simulink model "triplex_12B_with_contracts"  (R2019b)
settings: Solver=ode3  StartTime=0.0  StopTime=10.0  FixedStep=.1  RelTol=1e-3  EnableMultiTasking=on
model workspace (MAT data in the model file):
  ContractValidatorBlocksMap = containers.Map
  ContractValidatorBlocksMap.serialization.keys = {'triplex_12B/triplex_12B_TriplexSignalMonitorSpec/validator', 'triplex_12B_with_contracts/triplex_12B_TriplexSignalMonitorSpec/validator'}
  ContractValidatorBlocksMap.serialization.values{1}.block = 'triplex_12B/triplex_12B_TriplexSignalMonitorSpec/validator'
  ContractValidatorBlocksMap.serialization.values{1}.assumePorts = 1
  ContractValidatorBlocksMap.serialization.values{1}.guaranteePorts = 6
  ContractValidatorBlocksMap.serialization.values{1}.modeBlocksPorts = 0
  ContractValidatorBlocksMap.serialization.values{1}.portHandles.Inport = [1173.00195312 1174.00195312 1175.00195312 1176.00195312 1177.00195312 1178.00195312 1179.00195312]
  ContractValidatorBlocksMap.serialization.values{1}.portHandles.Outport = 1180.00195312
  ContractValidatorBlocksMap.serialization.values{1}.portHandles.Enable = []
  ContractValidatorBlocksMap.serialization.values{1}.portHandles.Trigger = []
  ContractValidatorBlocksMap.serialization.values{1}.portHandles.State = []
  ContractValidatorBlocksMap.serialization.values{1}.portHandles.LConn = []
  ContractValidatorBlocksMap.serialization.values{1}.portHandles.RConn = []
  ContractValidatorBlocksMap.serialization.values{1}.portHandles.Ifaction = []
  ContractValidatorBlocksMap.serialization.values{1}.portHandles.Reset = []
  ContractValidatorBlocksMap.serialization.values{1}.portConnectivity(1).Type = '1'
  ContractValidatorBlocksMap.serialization.values{1}.portConnectivity(1).Position = [365 -135]
  ContractValidatorBlocksMap.serialization.values{1}.portConnectivity(1).SrcBlock = 5288.00085449
  ContractValidatorBlocksMap.serialization.values{1}.portConnectivity(1).SrcPort = 0
  ContractValidatorBlocksMap.serialization.values{1}.portConnectivity(1).DstBlock = []
  ContractValidatorBlocksMap.serialization.values{1}.portConnectivity(1).DstPort = []
  ContractValidatorBlocksMap.serialization.values{1}.portConnectivity(2).Type = '2'
  ContractValidatorBlocksMap.serialization.values{1}.portConnectivity(2).Position = [365 -65]
  ContractValidatorBlocksMap.serialization.values{1}.portConnectivity(2).SrcBlock = 600.002807617
  ContractValidatorBlocksMap.serialization.values{1}.portConnectivity(2).SrcPort = 0
  ContractValidatorBlocksMap.serialization.values{1}.portConnectivity(2).DstBlock = []
  ContractValidatorBlocksMap.serialization.values{1}.portConnectivity(2).DstPort = []
  ContractValidatorBlocksMap.serialization.values{1}.portConnectivity(3).Type = '3'
  ContractValidatorBlocksMap.serialization.values{1}.portConnectivity(3).Position = [365 5]
  ContractValidatorBlocksMap.serialization.values{1}.portConnectivity(3).SrcBlock = 604.003051758
  ContractValidatorBlocksMap.serialization.values{1}.portConnectivity(3).SrcPort = 0
  ContractValidatorBlocksMap.serialization.values{1}.portConnectivity(3).DstBlock = []
  ContractValidatorBlocksMap.serialization.values{1}.portConnectivity(3).DstPort = []
  ContractValidatorBlocksMap.serialization.values{1}.portConnectivity(4).Type = '4'
  ContractValidatorBlocksMap.serialization.values{1}.portConnectivity(4).Position = [365 75]
  ContractValidatorBlocksMap.serialization.values{1}.portConnectivity(4).SrcBlock = 608.003051758
  ContractValidatorBlocksMap.serialization.values{1}.portConnectivity(4).SrcPort = 0
  ContractValidatorBlocksMap.serialization.values{1}.portConnectivity(4).DstBlock = []
  ContractValidatorBlocksMap.serialization.values{1}.portConnectivity(4).DstPort = []
  ContractValidatorBlocksMap.serialization.values{1}.portConnectivity(5).Type = '5'
  ContractValidatorBlocksMap.serialization.values{1}.portConnectivity(5).Position = [365 145]
  ContractValidatorBlocksMap.serialization.values{1}.portConnectivity(5).SrcBlock = 612.003051758
  ContractValidatorBlocksMap.serialization.values{1}.portConnectivity(5).SrcPort = 0
  ContractValidatorBlocksMap.serialization.values{1}.portConnectivity(5).DstBlock = []
  ContractValidatorBlocksMap.serialization.values{1}.portConnectivity(5).DstPort = []
  ContractValidatorBlocksMap.serialization.values{1}.portConnectivity(6).Type = '6'
  ContractValidatorBlocksMap.serialization.values{1}.portConnectivity(6).Position = [365 215]
  ContractValidatorBlocksMap.serialization.values{1}.portConnectivity(6).SrcBlock = 616.003051758
  ContractValidatorBlocksMap.serialization.values{1}.portConnectivity(6).SrcPort = 0
  ContractValidatorBlocksMap.serialization.values{1}.portConnectivity(6).DstBlock = []
  ContractValidatorBlocksMap.serialization.values{1}.portConnectivity(6).DstPort = []
  ContractValidatorBlocksMap.serialization.values{1}.portConnectivity(7).Type = '7'
  ContractValidatorBlocksMap.serialization.values{1}.portConnectivity(7).Position = [365 285]
  ContractValidatorBlocksMap.serialization.values{1}.portConnectivity(7).SrcBlock = 620.003051758
  ContractValidatorBlocksMap.serialization.values{1}.portConnectivity(7).SrcPort = 0
  ContractValidatorBlocksMap.serialization.values{1}.portConnectivity(7).DstBlock = []
  ContractValidatorBlocksMap.serialization.values{1}.portConnectivity(7).DstPort = []
  ContractValidatorBlocksMap.serialization.values{1}.portConnectivity(8).Type = '1'
  ContractValidatorBlocksMap.serialization.values{1}.portConnectivity(8).Position = [500 75]
  ContractValidatorBlocksMap.serialization.values{1}.portConnectivity(8).SrcBlock = []
  ContractValidatorBlocksMap.serialization.values{1}.portConnectivity(8).SrcPort = []
  ContractValidatorBlocksMap.serialization.values{1}.portConnectivity(8).DstBlock = 884.002807617
  ContractValidatorBlocksMap.serialization.values{1}.portConnectivity(8).DstPort = 0
  ContractValidatorBlocksMap.serialization.values{2}.block = 'triplex_12B_with_contracts/triplex_12B_TriplexSignalMonitorSpec/validator'
  ContractValidatorBlocksMap.serialization.values{2}.assumePorts = 0
  ContractValidatorBlocksMap.serialization.values{2}.guaranteePorts = 6
  ContractValidatorBlocksMap.serialization.values{2}.modeBlocksPorts = 0
  ContractValidatorBlocksMap.serialization.values{2}.portHandles.Inport = [2851.00183105 2852.00195312 2853.00195312 2854.00183105 2855.00195312 2856.00183105]
  ContractValidatorBlocksMap.serialization.values{2}.portHandles.Outport = 2857.00195312
  ContractValidatorBlocksMap.serialization.values{2}.portHandles.Enable = []
  ContractValidatorBlocksMap.serialization.values{2}.portHandles.Trigger = []
  ContractValidatorBlocksMap.serialization.values{2}.portHandles.State = []
  ContractValidatorBlocksMap.serialization.values{2}.portHandles.LConn = []
  ContractValidatorBlocksMap.serialization.values{2}.portHandles.RConn = []
  ContractValidatorBlocksMap.serialization.values{2}.portHandles.Ifaction = []
  ContractValidatorBlocksMap.serialization.values{2}.portHandles.Reset = []
  ContractValidatorBlocksMap.serialization.values{2}.portConnectivity(1).Type = '1'
  ContractValidatorBlocksMap.serialization.values{2}.portConnectivity(1).Position = [14780 -135]
  ContractValidatorBlocksMap.serialization.values{2}.portConnectivity(1).SrcBlock = 1475.00390625
  ContractValidatorBlocksMap.serialization.values{2}.portConnectivity(1).SrcPort = 0
  ContractValidatorBlocksMap.serialization.values{2}.portConnectivity(1).DstBlock = []
  ContractValidatorBlocksMap.serialization.values{2}.portConnectivity(1).DstPort = []
  ContractValidatorBlocksMap.serialization.values{2}.portConnectivity(2).Type = '2'
  ContractValidatorBlocksMap.serialization.values{2}.portConnectivity(2).Position = [14780 -50]
  ContractValidatorBlocksMap.serialization.values{2}.portConnectivity(2).SrcBlock = 1479.00378418
  ContractValidatorBlocksMap.serialization.values{2}.portConnectivity(2).SrcPort = 0
  ContractValidatorBlocksMap.serialization.values{2}.portConnectivity(2).DstBlock = []
  ContractValidatorBlocksMap.serialization.values{2}.portConnectivity(2).DstPort = []
  ContractValidatorBlocksMap.serialization.values{2}.portConnectivity(3).Type = '3'
  ContractValidatorBlocksMap.serialization.values{2}.portConnectivity(3).Position = [14780 35]
  ContractValidatorBlocksMap.serialization.values{2}.portConnectivity(3).SrcBlock = 1483.00402832
  ContractValidatorBlocksMap.serialization.values{2}.portConnectivity(3).SrcPort = 0
  ContractValidatorBlocksMap.serialization.values{2}.portConnectivity(3).DstBlock = []
  ContractValidatorBlocksMap.serialization.values{2}.portConnectivity(3).DstPort = []
  ContractValidatorBlocksMap.serialization.values{2}.portConnectivity(4).Type = '4'
  ContractValidatorBlocksMap.serialization.values{2}.portConnectivity(4).Position = [14780 120]
  ContractValidatorBlocksMap.serialization.values{2}.portConnectivity(4).SrcBlock = 1487.00354004
  ContractValidatorBlocksMap.serialization.values{2}.portConnectivity(4).SrcPort = 0
  ContractValidatorBlocksMap.serialization.values{2}.portConnectivity(4).DstBlock = []
  ContractValidatorBlocksMap.serialization.values{2}.portConnectivity(4).DstPort = []
  ContractValidatorBlocksMap.serialization.values{2}.portConnectivity(5).Type = '5'
  ContractValidatorBlocksMap.serialization.values{2}.portConnectivity(5).Position = [14780 205]
  ContractValidatorBlocksMap.serialization.values{2}.portConnectivity(5).SrcBlock = 1491.00524902
  ContractValidatorBlocksMap.serialization.values{2}.portConnectivity(5).SrcPort = 0
  ContractValidatorBlocksMap.serialization.values{2}.portConnectivity(5).DstBlock = []
  ContractValidatorBlocksMap.serialization.values{2}.portConnectivity(5).DstPort = []
  ContractValidatorBlocksMap.serialization.values{2}.portConnectivity(6).Type = '6'
  ContractValidatorBlocksMap.serialization.values{2}.portConnectivity(6).Position = [14780 290]
  ContractValidatorBlocksMap.serialization.values{2}.portConnectivity(6).SrcBlock = 1495.00378418
  ContractValidatorBlocksMap.serialization.values{2}.portConnectivity(6).SrcPort = 0
  ContractValidatorBlocksMap.serialization.values{2}.portConnectivity(6).DstBlock = []
  ContractValidatorBlocksMap.serialization.values{2}.portConnectivity(6).DstPort = []
  ContractValidatorBlocksMap.serialization.values{2}.portConnectivity(7).Type = '1'
  ContractValidatorBlocksMap.serialization.values{2}.portConnectivity(7).Position = [14915 80]
  ContractValidatorBlocksMap.serialization.values{2}.portConnectivity(7).SrcBlock = []
  ContractValidatorBlocksMap.serialization.values{2}.portConnectivity(7).SrcPort = []
  ContractValidatorBlocksMap.serialization.values{2}.portConnectivity(7).DstBlock = 2601.00195312
  ContractValidatorBlocksMap.serialization.values{2}.portConnectivity(7).DstPort = 0
  ContractValidatorBlocksMap.serialization.uniformity = 0
  ContractValidatorBlocksMap.serialization.keyType = 'char'
  ContractValidatorBlocksMap.serialization.valueType = 'any'
undefined symbols (not defined in the file): contractAfterSimulation, contractBeforeSimulation, ContractBlock, ContractGuaranteeBlock, ContractValidatorBlock, saveValidatorParameters
libraries: cocosimLibs x6
(part 1 of 2)
settings Model: Creator=elliocm  LastModifiedBy=hbourbou
settings DataIOCC: LimitDataPoints=on  SaveFormat=StructureWithTime  SignalLoggingSaveFormat=ModelDataLogs  ReturnWorkspaceOutputs=off
settings OptimizationCC: ExpressionDepthLimit=2147483647  LifeSpan=inf
settings DebuggingCC: UnderspecifiedInitializationDetection=Classic  MergeDetectMultiDrivingBlocksExec=none  SolverPrmCheckMsg=warning  MultiTaskDSMMsg=warning  MultiTaskCondExecSysMsg=none  StateNameClashWarn=warning  SFUnexpectedBacktrackingDiag=warning  SFNoUnconditionalDefaultTransitionDiag=warning  SFExecutionAtInitializationDiag=none  ArithmeticOperatorsInVariantConditions=warning
settings HardwareCC: ProdBitPerPointer=32  ProdBitPerSizeT=32  ProdBitPerPtrDiffT=32  ProdLargestAtomicFloat=None  ProdIntDivRoundTo=Undefined  ProdEndianess=Unspecified  ProdWordSize=32  ProdHWDeviceType=32-bit Generic
settings ModelReferenceCC: PropagateSignalLabelsOutOfModel=off
settings SFSimCC: SimUseLocalCustomCode=off  CustomCodeUndefinedFunction=UseInterfaceOnly
settings RTWCC: RTWUseLocalCustomCode=off
settings CodeAppCC: StateflowObjectComments=on
settings GRTTargetCC: TargetLangStandard=C89/C90 (ANSI)  GeneratePreprocessorConditionals=Disable all
settings ConfigComp: CovMetricSettings=dw  CovHtmlReporting=on  CovSaveCumulativeToWorkspaceVar=on  CovSaveSingleToWorkspaceVar=on  CovExternalEMLEnable=off

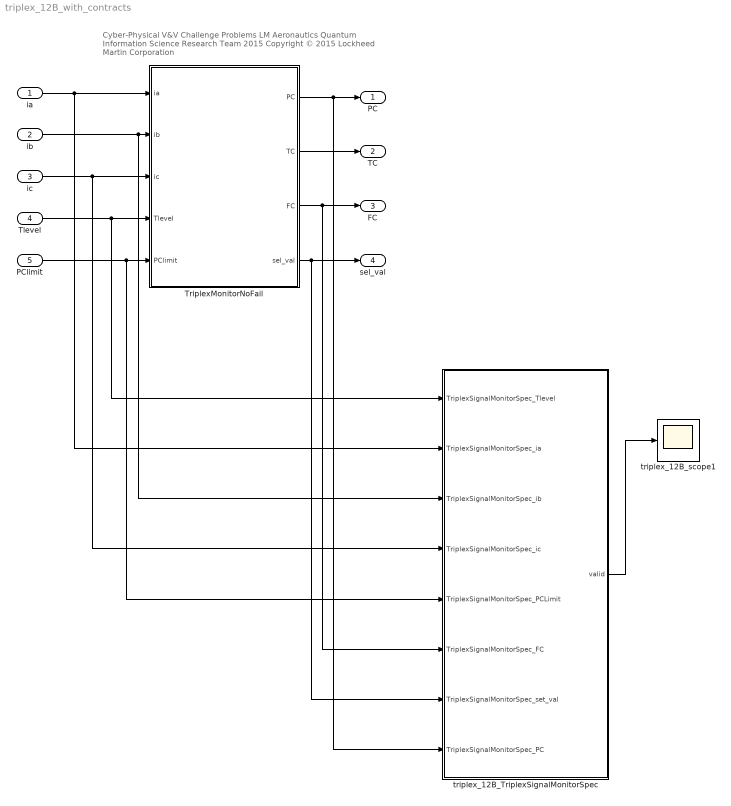
== system triplex_12B_with_contracts ==
  note: Cyber-Physical V&V Challenge Problems
      | LM Aeronautics Quantum Information Science Research Team 2015
      | Copyright © 2015 Lockheed Martin Corporation
  ia : Inport  OutDataTypeStr=double
  ib : Inport  Port=2  OutDataTypeStr=double
  ic : Inport  Port=3  OutDataTypeStr=double
  Tlevel : Inport  Port=4  OutDataTypeStr=double
  PClimit : Inport  Port=5  OutDataTypeStr=int32
  TriplexMonitorNoFail : Subsystem
  triplex_12B_TriplexSignalMonitorSpec : Subsystem  mask(ContractBlock){ContractBlockType=ContractBlock}
      mask init:
      | set_param(gcb, 'LinkStatus', 'none');
      mask DialogControl DescTextVar Prompt: Contract block
      mask Display:
      | text(0.5, 0.5, '{\bf\fontsize{20}Contract}', 'hor', 'center', 'texmode','on');
      | blocks = find_system(gcb, 'LookUnderMasks','all', 'SearchDepth',1,'BlockType','Inport');
      | for i = 1 : length(blocks)
      |     blockName = get_param(blocks(i), 'Name');
      |     [path, blockName] = fileparts(char(blockName));
      |     port_label('input', i, blockName);
      | end
      | 
      | blocks = find_system(gcb, 'LookUnderMasks','all', 'SearchDepth',1,'BlockType','Outport');
      | for i = 1 : length(blocks)
      |     blockName = get_param(blocks(i), 'Name');
      |     [path, blockName] = fileparts(char(blockName));
      |     port_label('output', i, blockName);
      | end
  triplex_12B_scope1 : Scope
  PC : Outport  VectorParamsAs1DForOutWhenUnconnected=off
  TC : Outport  Port=2  VectorParamsAs1DForOutWhenUnconnected=off
  FC : Outport  Port=3  VectorParamsAs1DForOutWhenUnconnected=off
  sel_val : Outport  Port=4  VectorParamsAs1DForOutWhenUnconnected=off
  wires:
  ia/1 -> TriplexMonitorNoFail/1(ia), triplex_12B_TriplexSignalMonitorSpec/2(TriplexSignalMonitorSpec_ia)
  ib/1 -> TriplexMonitorNoFail/2(ib), triplex_12B_TriplexSignalMonitorSpec/3(TriplexSignalMonitorSpec_ib)
  Tlevel/1 -> TriplexMonitorNoFail/4(Tlevel), triplex_12B_TriplexSignalMonitorSpec/1(TriplexSignalMonitorSpec_Tlevel)
  PClimit/1 -> TriplexMonitorNoFail/5(PClimit), triplex_12B_TriplexSignalMonitorSpec/5(TriplexSignalMonitorSpec_PCLimit)
  TriplexMonitorNoFail/2(TC) -> TC/1
  TriplexMonitorNoFail/1(PC) -> PC/1, triplex_12B_TriplexSignalMonitorSpec/8(TriplexSignalMonitorSpec_PC)
  TriplexMonitorNoFail/4(sel_val) -> sel_val/1, triplex_12B_TriplexSignalMonitorSpec/7(TriplexSignalMonitorSpec_set_val)
  ic/1 -> TriplexMonitorNoFail/3(ic), triplex_12B_TriplexSignalMonitorSpec/4(TriplexSignalMonitorSpec_ic)
  TriplexMonitorNoFail/3(FC) -> FC/1, triplex_12B_TriplexSignalMonitorSpec/6(TriplexSignalMonitorSpec_FC)
  triplex_12B_TriplexSignalMonitorSpec/1(valid) -> triplex_12B_scope1/1

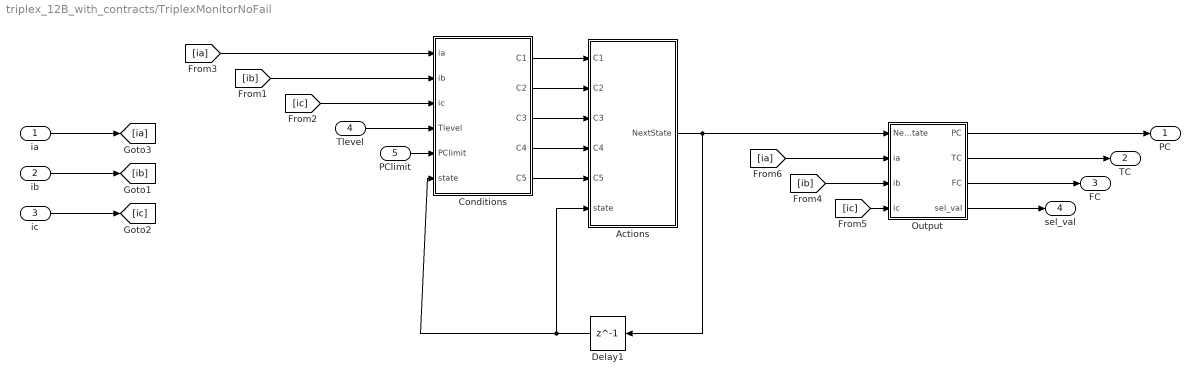
== system triplex_12B_with_contracts/TriplexMonitorNoFail ==
  ia : Inport
  ib : Inport  Port=2
  ic : Inport  Port=3
  Tlevel : Inport  Port=4
  PClimit : Inport  Port=5
  Actions : Subsystem
  Conditions : Subsystem
  Delay1 : Delay  DelayLength=1  InitialCondition=0
  Output : Subsystem
  PC : Outport  VectorParamsAs1DForOutWhenUnconnected=off
  TC : Outport  Port=2  VectorParamsAs1DForOutWhenUnconnected=off
  FC : Outport  Port=3  VectorParamsAs1DForOutWhenUnconnected=off
  sel_val : Outport  Port=4  VectorParamsAs1DForOutWhenUnconnected=off
  wires:
  Conditions/2(C2) -> Actions/2(C2)
  Conditions/5(C5) -> Actions/5(C5)
  Conditions/1(C1) -> Actions/1(C1)
  Conditions/4(C4) -> Actions/4(C4)
  Conditions/3(C3) -> Actions/3(C3)
  Tlevel/1 -> Conditions/4(Tlevel)
  PClimit/1 -> Conditions/5(PClimit)
  Output/2(TC) -> TC/1
  Output/1(PC) -> PC/1
  Output/3(FC) -> FC/1
  Actions/1(NextState) -> Delay1/1, Output/1(NextState)
  Delay1/1 -> Actions/6(state), Conditions/6(state)
  [ia] -> Conditions/1(ia)
  [ib] -> Conditions/2(ib)
  ia/1 -> [ia]
  ib/1 -> [ib]
  ic/1 -> [ic]
  [ic] -> Conditions/3(ic)
  [ia] -> Output/2(ia)
  [ib] -> Output/3(ib)
  [ic] -> Output/4(ic)
  Output/4(sel_val) -> sel_val/1

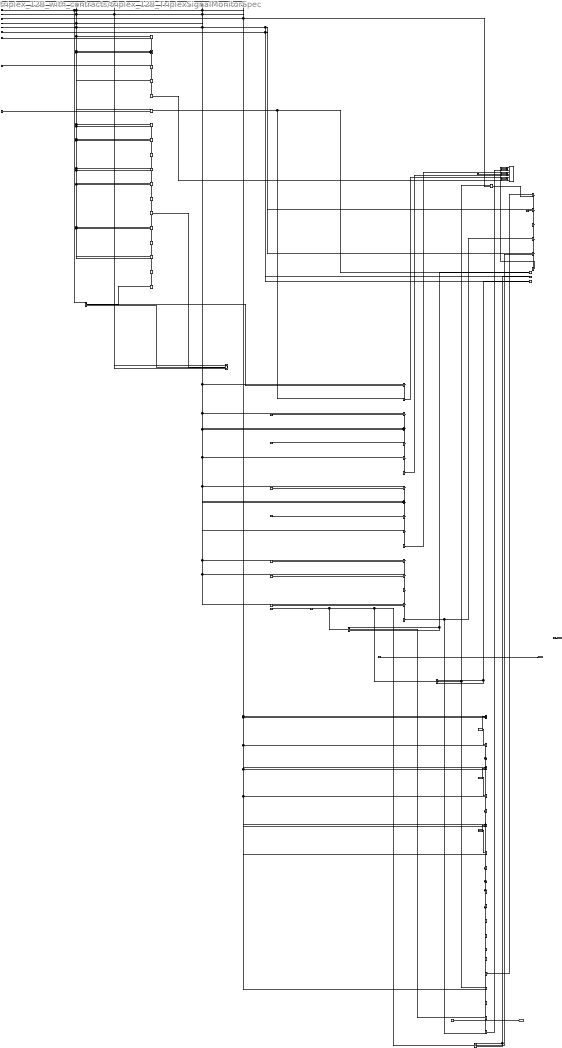
== system triplex_12B_with_contracts/triplex_12B_TriplexSignalMonitorSpec ==
  TriplexSignalMonitorSpec_Tlevel : Inport  OutDataTypeStr=double
  TriplexSignalMonitorSpec_ia : Inport  Port=2  OutDataTypeStr=double
  TriplexSignalMonitorSpec_ib : Inport  Port=3  OutDataTypeStr=double
  TriplexSignalMonitorSpec_ic : Inport  Port=4  OutDataTypeStr=double
  TriplexSignalMonitorSpec_PCLimit : Inport  Port=5
  TriplexSignalMonitorSpec_FC : Inport  Port=6
  TriplexSignalMonitorSpec_set_val : Inport  Port=7  OutDataTypeStr=double
  TriplexSignalMonitorSpec_PC : Inport  Port=8
  Arrow_xxTriplexS_443436564_ec_35_ni_0 : Delay  DelayLength=1  InitialCondition=1
  C1_operator : RelationalOperator  Operator=>  OutDataTypeStr=boolean  RndMeth=Simplest
  C2_operator : RelationalOperator  Operator=>  OutDataTypeStr=boolean  RndMeth=Simplest
  C3_operator : RelationalOperator  Operator=>  OutDataTypeStr=boolean  RndMeth=Simplest
  PRE_xxTriplexSignalMonitorSpec_37 : Delay  DelayLength=1  InitialCondition=0
  PRE_xxTriplexSignalMonitorSpec_40 : Delay  DelayLength=1  InitialCondition=0
  PRE_xxTriplexSignalMonitorSpec_46 : Delay  DelayLength=1  InitialCondition=0
  TSM-001 : Subsystem  mask(ContractGuaranteeBlock){ContractBlockType=ContractGuaranteeBlock}
      mask init:
      | set_param(gcb, 'LinkStatus', 'none');
      mask DialogControl DescTextVar Prompt: Guarantee block
  TSM-002 : Subsystem  mask(ContractGuaranteeBlock){ContractBlockType=ContractGuaranteeBlock}
      mask init:
      | set_param(gcb, 'LinkStatus', 'none');
      mask DialogControl DescTextVar Prompt: Guarantee block
  TSM-003a : Subsystem  mask(ContractGuaranteeBlock){ContractBlockType=ContractGuaranteeBlock}
      mask init:
      | set_param(gcb, 'LinkStatus', 'none');
      mask DialogControl DescTextVar Prompt: Guarantee block
  TSM-003b : Subsystem  mask(ContractGuaranteeBlock){ContractBlockType=ContractGuaranteeBlock}
      mask init:
      | set_param(gcb, 'LinkStatus', 'none');
      mask DialogControl DescTextVar Prompt: Guarantee block
  TSM-003c : Subsystem  mask(ContractGuaranteeBlock){ContractBlockType=ContractGuaranteeBlock}
      mask init:
      | set_param(gcb, 'LinkStatus', 'none');
      mask DialogControl DescTextVar Prompt: Guarantee block
  TSM-004 : Subsystem  mask(ContractGuaranteeBlock){ContractBlockType=ContractGuaranteeBlock}
      mask init:
      | set_param(gcb, 'LinkStatus', 'none');
      mask DialogControl DescTextVar Prompt: Guarantee block
  abs_call : Subsystem
  abs_call1 : Subsystem
  abs_call11 : Subsystem
  branch_10_IF : Switch  Criteria=u2 ~= 0
  branch_11_IF : Switch  Criteria=u2 ~= 0
  branch_12_IF : Switch  Criteria=u2 ~= 0
  branch_13_IF : Switch  Criteria=u2 ~= 0
  branch_9_IF : Switch  Criteria=u2 ~= 0
  failure_in_progress_operator : Logic  AllPortsSameDT=off  OutDataTypeStr=boolean
  failure_must_be_latched_operator : Logic  AllPortsSameDT=off  OutDataTypeStr=boolean
  miscompare_operator : Logic  Operator=OR  AllPortsSameDT=off  OutDataTypeStr=boolean
  no_fail_operator : RelationalOperator  Operator===  OutDataTypeStr=boolean  RndMeth=Simplest
  no_fail_rhs_2 : Constant  Value=0  OutDataTypeStr=int32
  single_fail_reported_operator : Logic  Operator=OR  AllPortsSameDT=off  OutDataTypeStr=boolean
  spec284_operator : cocosimLibs/Implies  SystemSampleTime=-1  Latency=0  AutoFrameSizeCalculation=off
  spec292_operator : cocosimLibs/Implies  SystemSampleTime=-1  Latency=0  AutoFrameSizeCalculation=off
  spec309_operator : cocosimLibs/Implies  SystemSampleTime=-1  Latency=0  AutoFrameSizeCalculation=off
  spec326_operator : cocosimLibs/Implies  SystemSampleTime=-1  Latency=0  AutoFrameSizeCalculation=off
  spec334_operator : cocosimLibs/Implies  SystemSampleTime=-1  Latency=0  AutoFrameSizeCalculation=off
  spec351_operator : cocosimLibs/Implies  SystemSampleTime=-1  Latency=0  AutoFrameSizeCalculation=off
  validator : M-S-Function  LoadFcn=saveValidatorParameters(gcb);  InitFcn=contractBeforeSimulation();  StopFcn=contractAfterSimulation();  FunctionName=contract  mask(ContractValidatorBlock){assumePorts=0, guaranteePorts=6, modePorts=0, ContractBlockType=ContractValidatorBlock, createInportsCheckbox=off}
      mask prompts: assumePorts "Assume ports     :"; guaranteePorts "Guarantee ports :"; modePorts "Mode ports        :"; createInportsCheckbox "Create inports and connect them automatically"
      mask init:
      | set_param(gcb,'LinkStatus','none');
      | contract_callback('inputs_callback',gcb);
      mask DialogControl DescTextVar Prompt: The validator block implements the following logic: <br> <br> <b>Sofar</b>(assume<sub>1</sub> <b>&#8743;</b> assume<sub>2</sub> <b>&#8743;</b> ... assume<sub>k</sub>) <b>&rarr;</b> (guarantee<sub>1</sub> <b>&#8743;</b> guarantee<sub>2</sub> <b>&#8743;</b> ... guarantee<sub>m</sub> <b>&#8743;</b>  mode<sub>1</sub> <b>&#8743;</b> mode<sub>2</sub> <b>&#8743;</b> ... <b>&#8743;</b> mode<sub>n</sub> )<br> where mode<sub>i</sub> = require<sub>i</sub> <b>&rarr;</b> ensure<sub>i</sub>
      mask Display:
      | color('black');
      | port_label('input',1,'guarantee');
      | port_label('input',2,'guarantee');
      | port_label('input',3,'guarantee');
      | port_label('input',4,'guarantee');
      | port_label('input',5,'guarantee');
      | port_label('input',6,'guarantee');
      | port_label('output',1,'valid');
  xxTriplexS_443436564_ec_35_ni_0_init : Constant  Value=0  OutDataTypeStr=boolean
  xxTriplexSignalMonitorSpec_10_operator : Sum  OutDataTypeStr=double
  xxTriplexSignalMonitorSpec_11_operator : Product  OutDataTypeStr=double
  xxTriplexSignalMonitorSpec_11_rhs_1 : Constant  Value=0.5  OutDataTypeStr=double
  xxTriplexSignalMonitorSpec_12_operator : RelationalOperator  Operator===  OutDataTypeStr=boolean  RndMeth=Simplest
  xxTriplexSignalMonitorSpec_13_operator : RelationalOperator  Operator===  OutDataTypeStr=boolean  RndMeth=Simplest
  xxTriplexSignalMonitorSpec_13_rhs_2 : Constant  Value=2  OutDataTypeStr=int32
  xxTriplexSignalMonitorSpec_14_operator : Logic  AllPortsSameDT=off  OutDataTypeStr=boolean
  xxTriplexSignalMonitorSpec_15_operator : RelationalOperator  Operator===  OutDataTypeStr=boolean  RndMeth=Simplest
  xxTriplexSignalMonitorSpec_16_operator : Logic  AllPortsSameDT=off  OutDataTypeStr=boolean
  xxTriplexSignalMonitorSpec_17_operator : Sum  Inputs=+-  OutDataTypeStr=double
  xxTriplexSignalMonitorSpec_19_operator : Sum  Inputs=+-  OutDataTypeStr=double
  xxTriplexSignalMonitorSpec_1_operator : Sum  OutDataTypeStr=double
  xxTriplexSignalMonitorSpec_21_operator : Sum  Inputs=+-  OutDataTypeStr=double
  xxTriplexSignalMonitorSpec_23_operator : RelationalOperator  Operator=<=  OutDataTypeStr=boolean  RndMeth=Simplest
  xxTriplexSignalMonitorSpec_24_operator : RelationalOperator  Operator=<=  OutDataTypeStr=boolean  RndMeth=Simplest
  xxTriplexSignalMonitorSpec_25_operator : Logic  AllPortsSameDT=off  OutDataTypeStr=boolean
  xxTriplexSignalMonitorSpec_26_operator : RelationalOperator  Operator=<=  OutDataTypeStr=boolean  RndMeth=Simplest
  xxTriplexSignalMonitorSpec_27_operator : RelationalOperator  Operator=<=  OutDataTypeStr=boolean  RndMeth=Simplest
  xxTriplexSignalMonitorSpec_28_operator : Logic  AllPortsSameDT=off  OutDataTypeStr=boolean
  xxTriplexSignalMonitorSpec_29_operator : Logic  Operator=OR  AllPortsSameDT=off  OutDataTypeStr=boolean
  xxTriplexSignalMonitorSpec_2_operator : Product  OutDataTypeStr=double
  xxTriplexSignalMonitorSpec_2_rhs_1 : Constant  Value=0.5  OutDataTypeStr=double
  xxTriplexSignalMonitorSpec_30_operator : RelationalOperator  Operator=<=  OutDataTypeStr=boolean  RndMeth=Simplest
  xxTriplexSignalMonitorSpec_31_operator : Logic  AllPortsSameDT=off  OutDataTypeStr=boolean
  xxTriplexSignalMonitorSpec_32_operator : RelationalOperator  Operator=<=  OutDataTypeStr=boolean  RndMeth=Simplest
  xxTriplexSignalMonitorSpec_33_operator : Logic  AllPortsSameDT=off  OutDataTypeStr=boolean
  xxTriplexSignalMonitorSpec_34_operator : Logic  Operator=OR  AllPortsSameDT=off  OutDataTypeStr=boolean
  xxTriplexSignalMonitorSpec_36_rhs : Constant  Value=0  OutDataTypeStr=Inherit: Inherit via back propagation
  xxTriplexSignalMonitorSpec_39_rhs : Constant  Value=0.0  OutDataTypeStr=double
  xxTriplexSignalMonitorSpec_3_operator : RelationalOperator  Operator===  OutDataTypeStr=boolean  RndMeth=Simplest
  xxTriplexSignalMonitorSpec_42_operator : RelationalOperator  Operator=>  OutDataTypeStr=boolean  RndMeth=Simplest
  xxTriplexSignalMonitorSpec_42_rhs_2 : Constant  Value=0  OutDataTypeStr=int32
  xxTriplexSignalMonitorSpec_43_operator : RelationalOperator  Operator=<=  OutDataTypeStr=boolean  RndMeth=Simplest
  xxTriplexSignalMonitorSpec_44_operator : Logic  AllPortsSameDT=off  OutDataTypeStr=boolean
  xxTriplexSignalMonitorSpec_45_operator : RelationalOperator  Operator=>  OutDataTypeStr=boolean  RndMeth=Simplest
  xxTriplexSignalMonitorSpec_47_rhs1 : Constant  Value=true  OutDataTypeStr=boolean
  xxTriplexSignalMonitorSpec_48_operator : RelationalOperator  Operator===  OutDataTypeStr=boolean  RndMeth=Simplest
  xxTriplexSignalMonitorSpec_48_rhs_2 : Constant  Value=4  OutDataTypeStr=int32
  xxTriplexSignalMonitorSpec_49_operator : RelationalOperator  Operator===  OutDataTypeStr=boolean  RndMeth=Simplest
  xxTriplexSignalMonitorSpec_49_rhs_2 : Constant  Value=2  OutDataTypeStr=int32
  xxTriplexSignalMonitorSpec_4_operator : RelationalOperator  Operator===  OutDataTypeStr=boolean  RndMeth=Simplest
  xxTriplexSignalMonitorSpec_4_rhs_2 : Constant  OutDataTypeStr=int32
  xxTriplexSignalMonitorSpec_50_operator : RelationalOperator  Operator===  OutDataTypeStr=boolean  RndMeth=Simplest
  xxTriplexSignalMonitorSpec_50_rhs_2 : Constant  OutDataTypeStr=int32
  xxTriplexSignalMonitorSpec_51_operator : Logic  Operator=OR  AllPortsSameDT=off  OutDataTypeStr=boolean
  xxTriplexSignalMonitorSpec_52_operator : Logic  Operator=NOT  AllPortsSameDT=off  OutDataTypeStr=boolean
  xxTriplexSignalMonitorSpec_53_operator : Logic  AllPortsSameDT=off  OutDataTypeStr=boolean
  xxTriplexSignalMonitorSpec_54_operator : Logic  AllPortsSameDT=off  OutDataTypeStr=boolean
  xxTriplexSignalMonitorSpec_55_operator : Logic  Operator=NOT  AllPortsSameDT=off  OutDataTypeStr=boolean
  xxTriplexSignalMonitorSpec_56_operator : Logic  AllPortsSameDT=off  OutDataTypeStr=boolean
  xxTriplexSignalMonitorSpec_57_operator : Logic  AllPortsSameDT=off  OutDataTypeStr=boolean
  xxTriplexSignalMonitorSpec_58_operator : Logic  Operator=NOT  AllPortsSameDT=off  OutDataTypeStr=boolean
  xxTriplexSignalMonitorSpec_59_operator : Logic  AllPortsSameDT=off  OutDataTypeStr=boolean
  xxTriplexSignalMonitorSpec_5_operator : RelationalOperator  Operator===  OutDataTypeStr=boolean  RndMeth=Simplest
  xxTriplexSignalMonitorSpec_60_operator : Logic  AllPortsSameDT=off  OutDataTypeStr=boolean
  xxTriplexSignalMonitorSpec_61_operator : Logic  Operator=OR  AllPortsSameDT=off  OutDataTypeStr=boolean
  xxTriplexSignalMonitorSpec_6_operator : Sum  OutDataTypeStr=double
  xxTriplexSignalMonitorSpec_7_operator : Product  OutDataTypeStr=double
  xxTriplexSignalMonitorSpec_7_rhs_1 : Constant  Value=0.5  OutDataTypeStr=double
  xxTriplexSignalMonitorSpec_8_operator : RelationalOperator  Operator===  OutDataTypeStr=boolean  RndMeth=Simplest
  xxTriplexSignalMonitorSpec_9_operator : RelationalOperator  Operator===  OutDataTypeStr=boolean  RndMeth=Simplest
  xxTriplexSignalMonitorSpec_9_rhs_2 : Constant  Value=4  OutDataTypeStr=int32
  valid : Outport
  wires:
  validator/1 -> valid/1
  xxTriplexSignalMonitorSpec_9_rhs_2/1 -> xxTriplexSignalMonitorSpec_9_operator/2
  xxTriplexSignalMonitorSpec_7_operator/1 -> xxTriplexSignalMonitorSpec_8_operator/2
  xxTriplexSignalMonitorSpec_6_operator/1 -> xxTriplexSignalMonitorSpec_7_operator/2
  xxTriplexSignalMonitorSpec_7_rhs_1/1 -> xxTriplexSignalMonitorSpec_7_operator/1
  xxTriplexSignalMonitorSpec_57_operator/1 -> xxTriplexSignalMonitorSpec_61_operator/2
  xxTriplexSignalMonitorSpec_60_operator/1 -> xxTriplexSignalMonitorSpec_61_operator/1
  xxTriplexSignalMonitorSpec_59_operator/1 -> xxTriplexSignalMonitorSpec_60_operator/1
  branch_9_IF/1 -> xxTriplexSignalMonitorSpec_5_operator/2
  xxTriplexSignalMonitorSpec_58_operator/1 -> xxTriplexSignalMonitorSpec_59_operator/1
  xxTriplexSignalMonitorSpec_56_operator/1 -> xxTriplexSignalMonitorSpec_57_operator/1
  xxTriplexSignalMonitorSpec_55_operator/1 -> xxTriplexSignalMonitorSpec_56_operator/2
  xxTriplexSignalMonitorSpec_52_operator/1 -> xxTriplexSignalMonitorSpec_54_operator/2
  xxTriplexSignalMonitorSpec_53_operator/1 -> xxTriplexSignalMonitorSpec_54_operator/1
  xxTriplexSignalMonitorSpec_49_operator/1 -> xxTriplexSignalMonitorSpec_51_operator/2
  xxTriplexSignalMonitorSpec_50_operator/1 -> xxTriplexSignalMonitorSpec_51_operator/1
  xxTriplexSignalMonitorSpec_50_rhs_2/1 -> xxTriplexSignalMonitorSpec_50_operator/2
  xxTriplexSignalMonitorSpec_4_rhs_2/1 -> xxTriplexSignalMonitorSpec_4_operator/2
  xxTriplexSignalMonitorSpec_49_rhs_2/1 -> xxTriplexSignalMonitorSpec_49_operator/2
  xxTriplexSignalMonitorSpec_48_rhs_2/1 -> xxTriplexSignalMonitorSpec_48_operator/2
  xxTriplexSignalMonitorSpec_47_rhs1/1 -> [a_e_xxTriplexSignalMonitorSpec_47]
  xxTriplexSignalMonitorSpec_43_operator/1 -> xxTriplexSignalMonitorSpec_44_operator/2
  xxTriplexSignalMonitorSpec_42_rhs_2/1 -> xxTriplexSignalMonitorSpec_42_operator/2
  xxTriplexSignalMonitorSpec_39_rhs/1 -> [a_e_xxTriplexSignalMonitorSpec_41]
  xxTriplexSignalMonitorSpec_2_operator/1 -> xxTriplexSignalMonitorSpec_3_operator/2
  xxTriplexSignalMonitorSpec_36_rhs/1 -> [a_e_xxTriplexSignalMonitorSpec_38]
  xxTriplexSignalMonitorSpec_31_operator/1 -> xxTriplexSignalMonitorSpec_34_operator/2
  xxTriplexSignalMonitorSpec_33_operator/1 -> xxTriplexSignalMonitorSpec_34_operator/1
  xxTriplexSignalMonitorSpec_32_operator/1 -> xxTriplexSignalMonitorSpec_33_operator/2
  xxTriplexSignalMonitorSpec_30_operator/1 -> xxTriplexSignalMonitorSpec_31_operator/1
  xxTriplexSignalMonitorSpec_1_operator/1 -> xxTriplexSignalMonitorSpec_2_operator/2
  xxTriplexSignalMonitorSpec_2_rhs_1/1 -> xxTriplexSignalMonitorSpec_2_operator/1
  xxTriplexSignalMonitorSpec_25_operator/1 -> xxTriplexSignalMonitorSpec_29_operator/2
  xxTriplexSignalMonitorSpec_28_operator/1 -> xxTriplexSignalMonitorSpec_29_operator/1
  xxTriplexSignalMonitorSpec_26_operator/1 -> xxTriplexSignalMonitorSpec_28_operator/2
  xxTriplexSignalMonitorSpec_24_operator/1 -> xxTriplexSignalMonitorSpec_25_operator/1
  failure_in_progress_operator/1 -> xxTriplexSignalMonitorSpec_16_operator/2
  branch_13_IF/1 -> xxTriplexSignalMonitorSpec_15_operator/2
  failure_must_be_latched_operator/1 -> xxTriplexSignalMonitorSpec_14_operator/2
  branch_11_IF/1 -> xxTriplexSignalMonitorSpec_14_operator/1
  xxTriplexSignalMonitorSpec_13_rhs_2/1 -> xxTriplexSignalMonitorSpec_13_operator/2
  xxTriplexSignalMonitorSpec_11_operator/1 -> xxTriplexSignalMonitorSpec_12_operator/2
  xxTriplexSignalMonitorSpec_10_operator/1 -> xxTriplexSignalMonitorSpec_11_operator/2
  xxTriplexSignalMonitorSpec_11_rhs_1/1 -> xxTriplexSignalMonitorSpec_11_operator/1
  TSM-003a/1(guarantee) -> validator/6
  TSM-002/1(guarantee) -> validator/5
  TSM-003c/1(guarantee) -> validator/4
  TSM-003b/1(guarantee) -> validator/3
  TSM-001/1(guarantee) -> validator/2
  TSM-004/1(guarantee) -> validator/1
  xxTriplexSignalMonitorSpec_3_operator/1 -> spec351_operator/2
  xxTriplexSignalMonitorSpec_4_operator/1 -> spec351_operator/1
  xxTriplexSignalMonitorSpec_5_operator/1 -> spec334_operator/2
  xxTriplexSignalMonitorSpec_8_operator/1 -> spec326_operator/2
  xxTriplexSignalMonitorSpec_9_operator/1 -> spec326_operator/1
  xxTriplexSignalMonitorSpec_12_operator/1 -> spec309_operator/2
  xxTriplexSignalMonitorSpec_13_operator/1 -> spec309_operator/1
  xxTriplexSignalMonitorSpec_14_operator/1 -> spec292_operator/1
  xxTriplexSignalMonitorSpec_15_operator/1 -> spec284_operator/2
  xxTriplexSignalMonitorSpec_16_operator/1 -> spec284_operator/1
  xxTriplexSignalMonitorSpec_48_operator/1 -> single_fail_reported_operator/2
  xxTriplexSignalMonitorSpec_51_operator/1 -> single_fail_reported_operator/1
  no_fail_rhs_2/1 -> no_fail_operator/2
  xxTriplexSignalMonitorSpec_54_operator/1 -> miscompare_operator/2
  xxTriplexSignalMonitorSpec_61_operator/1 -> miscompare_operator/1
  spec351_operator/1 -> TSM-003a/1(In1)
  spec334_operator/1 -> TSM-002/1(In1)
  spec326_operator/1 -> TSM-003c/1(In1)
  spec309_operator/1 -> TSM-003b/1(In1)
  spec292_operator/1 -> TSM-001/1(In1)
  spec284_operator/1 -> TSM-004/1(In1)
  xxTriplexSignalMonitorSpec_45_operator/1 -> failure_must_be_latched_operator/2
  xxTriplexSignalMonitorSpec_42_operator/1 -> failure_in_progress_operator/2
  xxTriplexSignalMonitorSpec_44_operator/1 -> failure_in_progress_operator/1
  branch_10_IF/1 -> branch_9_IF/3
  xxTriplexSignalMonitorSpec_29_operator/1 -> branch_9_IF/2
  xxTriplexSignalMonitorSpec_34_operator/1 -> branch_10_IF/2
  xxTriplexSignalMonitorSpec_21_operator/1 -> abs_call11/1(abs_x)
  xxTriplexSignalMonitorSpec_19_operator/1 -> abs_call1/1(abs_x)
  xxTriplexSignalMonitorSpec_17_operator/1 -> abs_call/1(abs_x)
  abs_call11/1(abs_y) -> C3_operator/1
  abs_call1/1(abs_y) -> C2_operator/1
  abs_call/1(abs_y) -> C1_operator/1
  xxTriplexS_443436564_ec_35_ni_0_init/1 -> Arrow_xxTriplexS_443436564_ec_35_ni_0/1
  TriplexSignalMonitorSpec_PC/1 -> xxTriplexSignalMonitorSpec_42_operator/1, PRE_xxTriplexSignalMonitorSpec_37/1
  TriplexSignalMonitorSpec_PCLimit/1 -> xxTriplexSignalMonitorSpec_45_operator/2, xxTriplexSignalMonitorSpec_43_operator/2
  branch_12_IF/1 -> xxTriplexSignalMonitorSpec_45_operator/1, xxTriplexSignalMonitorSpec_43_operator/1
  PRE_xxTriplexSignalMonitorSpec_40/1 -> branch_13_IF/3, branch_13_IF/1
  single_fail_reported_operator/1 -> xxTriplexSignalMonitorSpec_16_operator/1, spec292_operator/2
  miscompare_operator/1 -> xxTriplexSignalMonitorSpec_44_operator/1, failure_must_be_latched_operator/1
  C3_operator/1 -> xxTriplexSignalMonitorSpec_57_operator/2, xxTriplexSignalMonitorSpec_52_operator/1, xxTriplexSignalMonitorSpec_60_operator/2
  C2_operator/1 -> xxTriplexSignalMonitorSpec_55_operator/1, xxTriplexSignalMonitorSpec_53_operator/2, xxTriplexSignalMonitorSpec_59_operator/2
  C1_operator/1 -> xxTriplexSignalMonitorSpec_56_operator/1, xxTriplexSignalMonitorSpec_53_operator/1, xxTriplexSignalMonitorSpec_58_operator/1
  TriplexSignalMonitorSpec_Tlevel/1 -> C3_operator/2, C2_operator/2, C1_operator/2
  PRE_xxTriplexSignalMonitorSpec_37/1 -> branch_12_IF/3, branch_12_IF/1
  Arrow_xxTriplexS_443436564_ec_35_ni_0/1 -> branch_13_IF/2, branch_12_IF/2, branch_11_IF/2
  PRE_xxTriplexSignalMonitorSpec_46/1 -> branch_11_IF/3, branch_11_IF/1
  TriplexSignalMonitorSpec_set_val/1 -> xxTriplexSignalMonitorSpec_8_operator/1, xxTriplexSignalMonitorSpec_12_operator/1, xxTriplexSignalMonitorSpec_5_operator/1, xxTriplexSignalMonitorSpec_15_operator/1, PRE_xxTriplexSignalMonitorSpec_40/1, xxTriplexSignalMonitorSpec_3_operator/1
  no_fail_operator/1 -> spec334_operator/1, PRE_xxTriplexSignalMonitorSpec_46/1
  TriplexSignalMonitorSpec_ia/1 -> xxTriplexSignalMonitorSpec_30_operator/2, xxTriplexSignalMonitorSpec_27_operator/1, xxTriplexSignalMonitorSpec_23_operator/2, xxTriplexSignalMonitorSpec_32_operator/1, xxTriplexSignalMonitorSpec_1_operator/1, xxTriplexSignalMonitorSpec_21_operator/1, xxTriplexSignalMonitorSpec_17_operator/1, xxTriplexSignalMonitorSpec_10_operator/1, branch_10_IF/1
  TriplexSignalMonitorSpec_ib/1 -> xxTriplexSignalMonitorSpec_26_operator/1, xxTriplexSignalMonitorSpec_24_operator/2, xxTriplexSignalMonitorSpec_27_operator/2, xxTriplexSignalMonitorSpec_23_operator/1, xxTriplexSignalMonitorSpec_1_operator/2, xxTriplexSignalMonitorSpec_19_operator/1, xxTriplexSignalMonitorSpec_17_operator/2, xxTriplexSignalMonitorSpec_6_operator/1, branch_9_IF/1
  TriplexSignalMonitorSpec_ic/1 -> xxTriplexSignalMonitorSpec_26_operator/2, xxTriplexSignalMonitorSpec_24_operator/1, xxTriplexSignalMonitorSpec_30_operator/1, xxTriplexSignalMonitorSpec_32_operator/2, xxTriplexSignalMonitorSpec_6_operator/2, xxTriplexSignalMonitorSpec_10_operator/2, xxTriplexSignalMonitorSpec_21_operator/2, xxTriplexSignalMonitorSpec_19_operator/2, branch_10_IF/3
  xxTriplexSignalMonitorSpec_23_operator/1 -> xxTriplexSignalMonitorSpec_33_operator/1, xxTriplexSignalMonitorSpec_25_operator/2
  xxTriplexSignalMonitorSpec_27_operator/1 -> xxTriplexSignalMonitorSpec_31_operator/2, xxTriplexSignalMonitorSpec_28_operator/1
  TriplexSignalMonitorSpec_FC/1 -> xxTriplexSignalMonitorSpec_4_operator/1, no_fail_operator/1, xxTriplexSignalMonitorSpec_49_operator/1, xxTriplexSignalMonitorSpec_48_operator/1, xxTriplexSignalMonitorSpec_50_operator/1, xxTriplexSignalMonitorSpec_13_operator/1, xxTriplexSignalMonitorSpec_9_operator/1

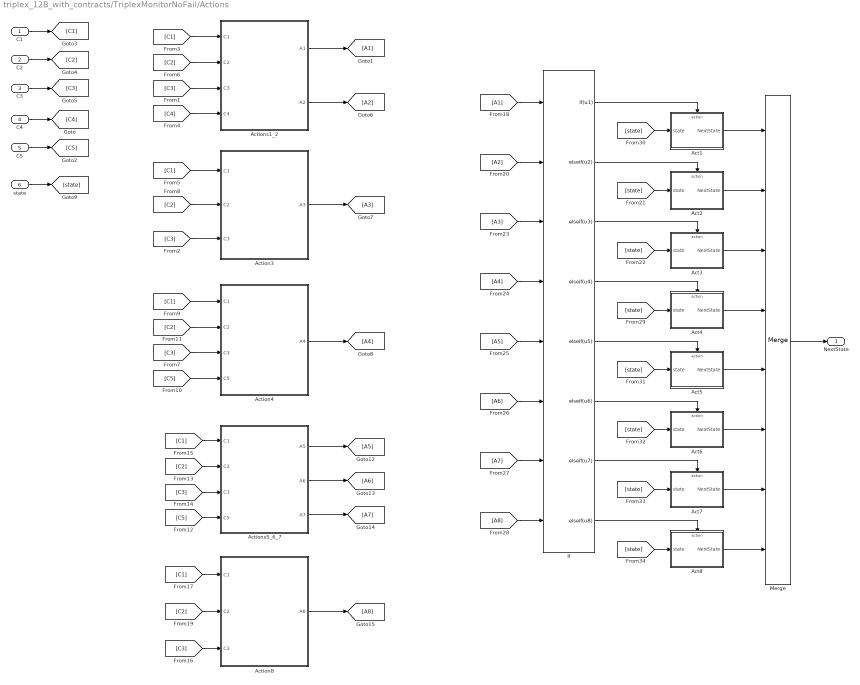
== system triplex_12B_with_contracts/TriplexMonitorNoFail/Actions ==
  C1 : Inport
  C2 : Inport  Port=2
  C3 : Inport  Port=3
  C4 : Inport  Port=4
  C5 : Inport  Port=5
  state : Inport  Port=6
  Act1 : Subsystem
  Act2 : Subsystem
  Act3 : Subsystem
  Act4 : Subsystem
  Act5 : Subsystem
  Act6 : Subsystem
  Act7 : Subsystem
  Act8 : Subsystem
  Action3 : Subsystem
  Action4 : Subsystem
  Action8 : Subsystem
  Actions1_2 : Subsystem
  Actions5_6_7 : Subsystem
  If : If  NumInputs=8  IfExpression=u1  ElseIfExpressions=u2, u3, u4, u5, u6, u7, u8  ShowElse=off
  Merge : Merge  Inputs=8
  NextState : Outport  VectorParamsAs1DForOutWhenUnconnected=off
  wires:
  C1/1 -> [C1]
  C5/1 -> [C5]
  C2/1 -> [C2]
  C3/1 -> [C3]
  C4/1 -> [C4]
  [C1] -> Actions1_2/1(C1)
  [C2] -> Actions1_2/2(C2)
  [C4] -> Actions1_2/4(C4)
  [C3] -> Actions1_2/3(C3)
  Actions1_2/2(A2) -> [A2]
  [C1] -> Action3/1(C1)
  [C2] -> Action3/2(C2)
  [C3] -> Action3/3(C3)
  Action4/1(A4) -> [A4]
  [C1] -> Action4/1(C1)
  [C2] -> Action4/2(C2)
  [C3] -> Action4/3(C3)
  [C5] -> Action4/4(C5)
  [C2] -> Actions5_6_7/2(C2)
  [C3] -> Actions5_6_7/3(C3)
  [C1] -> Actions5_6_7/1(C1)
  [C5] -> Actions5_6_7/4(C5)
  [C1] -> Action8/1(C1)
  [C2] -> Action8/2(C2)
  [C3] -> Action8/3(C3)
  Actions1_2/1(A1) -> [A1]
  Action3/1(A3) -> [A3]
  [A1] -> If/1
  If/1 -> Act1/Action
  [A2] -> If/2
  state/1 -> [state]
  If/2 -> Act2/Action
  If/3 -> Act3/Action
  [A3] -> If/3
  [A4] -> If/4
  [A5] -> If/5
  [A6] -> If/6
  [A7] -> If/7
  [A8] -> If/8
  If/4 -> Act4/Action
  Actions5_6_7/1(A5) -> [A5]
  Actions5_6_7/2(A6) -> [A6]
  Actions5_6_7/3(A7) -> [A7]
  Action8/1(A8) -> [A8]
  [state] -> Act1/1(state)
  If/5 -> Act5/Action
  If/6 -> Act6/Action
  If/7 -> Act7/Action
  If/8 -> Act8/Action
  Act1/1(NextState) -> Merge/1
  Act2/1(NextState) -> Merge/2
  Act3/1(NextState) -> Merge/3
  Act4/1(NextState) -> Merge/4
  Act5/1(NextState) -> Merge/5
  Act6/1(NextState) -> Merge/6
  Act7/1(NextState) -> Merge/7
  Act8/1(NextState) -> Merge/8
  Merge/1 -> NextState/1
  [state] -> Act2/1(state)
  [state] -> Act3/1(state)
  [state] -> Act4/1(state)
  [state] -> Act5/1(state)
  [state] -> Act6/1(state)
  [state] -> Act7/1(state)
  [state] -> Act8/1(state)

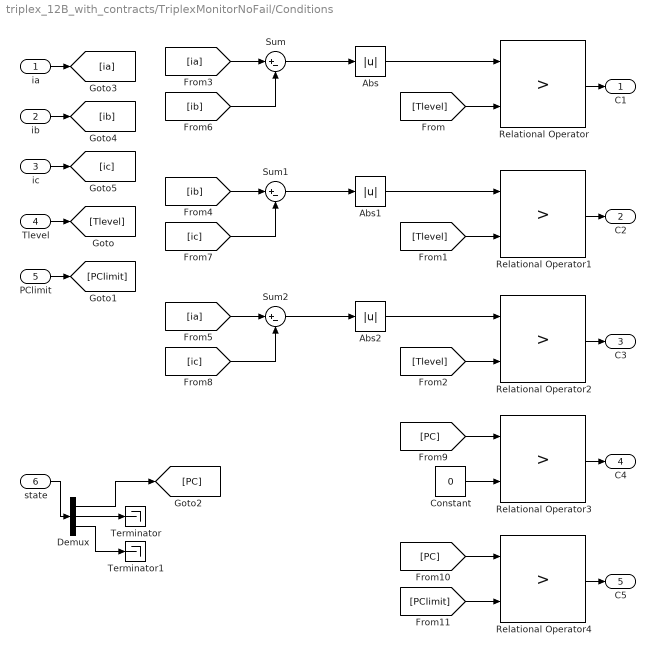
== system triplex_12B_with_contracts/TriplexMonitorNoFail/Conditions ==
  ia : Inport
  ib : Inport  Port=2
  ic : Inport  Port=3
  Tlevel : Inport  Port=4
  PClimit : Inport  Port=5
  state : Inport  Port=6
  Abs : Abs
  Abs1 : Abs
  Abs2 : Abs
  Constant : Constant  Value=0
  Demux : Demux  Outputs=3
  Relational Operator{,1..4} (5 alike) : RelationalOperator  Operator=>  OutDataTypeStr=boolean  RndMeth=Nearest
  Sum : Sum  Inputs=|+-
  Sum1 : Sum  Inputs=|+-
  Sum2 : Sum  Inputs=|+-
  Terminator : Terminator
  Terminator1 : Terminator
  C1 : Outport  VectorParamsAs1DForOutWhenUnconnected=off
  C2 : Outport  Port=2  VectorParamsAs1DForOutWhenUnconnected=off
  C3 : Outport  Port=3  VectorParamsAs1DForOutWhenUnconnected=off
  C4 : Outport  Port=4  VectorParamsAs1DForOutWhenUnconnected=off
  C5 : Outport  Port=5  VectorParamsAs1DForOutWhenUnconnected=off
  wires:
  Abs/1 -> Relational Operator/1
  Sum/1 -> Abs/1
  [Tlevel] -> Relational Operator/2
  Constant/1 -> Relational Operator3/2
  Abs1/1 -> Relational Operator1/1
  [Tlevel] -> Relational Operator1/2
  Sum1/1 -> Abs1/1
  Sum2/1 -> Abs2/1
  Abs2/1 -> Relational Operator2/1
  [Tlevel] -> Relational Operator2/2
  Relational Operator4/1 -> C5/1
  ib/1 -> [ib]
  [ia] -> Sum/1
  Relational Operator1/1 -> C2/1
  [PC] -> Relational Operator4/1
  Tlevel/1 -> [Tlevel]
  [ic] -> Sum1/2
  ia/1 -> [ia]
  ic/1 -> [ic]
  Relational Operator2/1 -> C3/1
  [ic] -> Sum2/2
  [ia] -> Sum2/1
  [ib] -> Sum/2
  [ib] -> Sum1/1
  [PC] -> Relational Operator3/1
  Relational Operator3/1 -> C4/1
  [PClimit] -> Relational Operator4/2
  PClimit/1 -> [PClimit]
  Relational Operator/1 -> C1/1
  state/1 -> Demux/1
  Demux/1 -> [PC]
  Demux/2 -> Terminator/1
  Demux/3 -> Terminator1/1

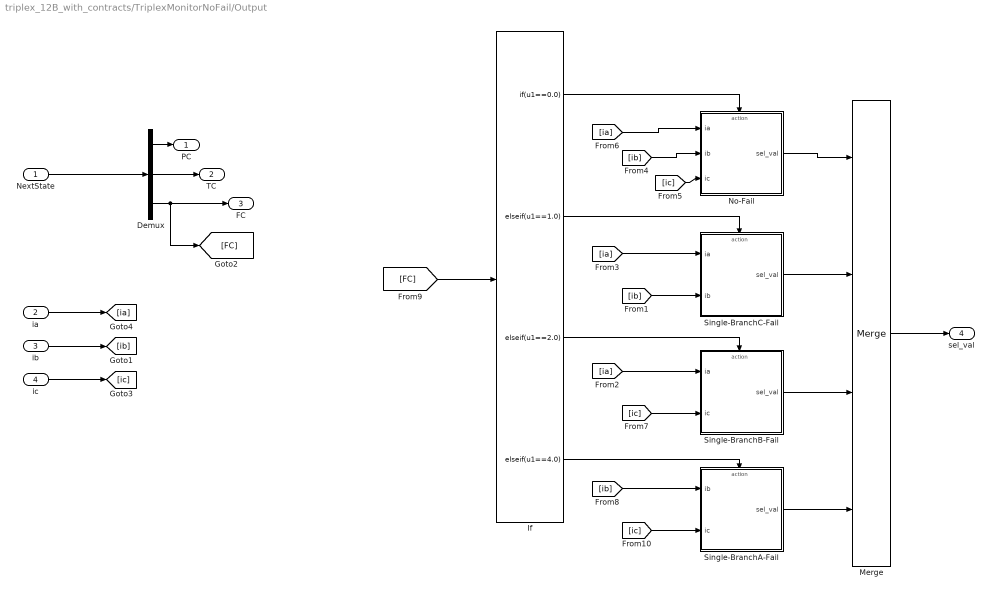
== system triplex_12B_with_contracts/TriplexMonitorNoFail/Output ==
  NextState : Inport
  ia : Inport  Port=2
  ib : Inport  Port=3
  ic : Inport  Port=4
  Demux : Demux  Outputs=3
  If : If  IfExpression=u1==0.0  ElseIfExpressions=u1==1.0, u1==2.0, u1==4.0  ShowElse=off
  Merge : Merge  Inputs=4
  No-Fail : Subsystem
  Single-BranchA-Fail : Subsystem
  Single-BranchB-Fail : Subsystem
  Single-BranchC-Fail : Subsystem
  PC : Outport  VectorParamsAs1DForOutWhenUnconnected=off
  TC : Outport  Port=2  VectorParamsAs1DForOutWhenUnconnected=off
  FC : Outport  Port=3  VectorParamsAs1DForOutWhenUnconnected=off
  sel_val : Outport  Port=4  VectorParamsAs1DForOutWhenUnconnected=off
  wires:
  NextState/1 -> Demux/1
  Demux/1 -> PC/1
  Demux/2 -> TC/1
  Demux/3 -> [FC], FC/1
  [FC] -> If/1
  If/1 -> No-Fail/Action
  ia/1 -> [ia]
  ib/1 -> [ib]
  ic/1 -> [ic]
  Merge/1 -> sel_val/1
  [ia] -> No-Fail/1(ia)
  [ib] -> No-Fail/2(ib)
  [ic] -> No-Fail/3(ic)
  If/2 -> Single-BranchC-Fail/Action
  [ia] -> Single-BranchC-Fail/1(ia)
  [ib] -> Single-BranchC-Fail/2(ib)
  If/3 -> Single-BranchB-Fail/Action
  [ia] -> Single-BranchB-Fail/1(ia)
  [ic] -> Single-BranchB-Fail/2(ic)
  If/4 -> Single-BranchA-Fail/Action
  [ib] -> Single-BranchA-Fail/1(ib)
  [ic] -> Single-BranchA-Fail/2(ic)
  No-Fail/1(sel_val) -> Merge/1
  Single-BranchC-Fail/1(sel_val) -> Merge/2
  Single-BranchB-Fail/1(sel_val) -> Merge/3
  Single-BranchA-Fail/1(sel_val) -> Merge/4

== system triplex_12B_with_contracts/triplex_12B_TriplexSignalMonitorSpec/TSM-001 ==
  In1 : Inport
  guarantee : Outport  OutDataTypeStr=boolean
  wires:
  In1/1 -> guarantee/1

== system triplex_12B_with_contracts/triplex_12B_TriplexSignalMonitorSpec/TSM-002 ==
  In1 : Inport
  guarantee : Outport  OutDataTypeStr=boolean
  wires:
  In1/1 -> guarantee/1

== system triplex_12B_with_contracts/triplex_12B_TriplexSignalMonitorSpec/TSM-003a ==
  In1 : Inport
  guarantee : Outport  OutDataTypeStr=boolean
  wires:
  In1/1 -> guarantee/1

== system triplex_12B_with_contracts/triplex_12B_TriplexSignalMonitorSpec/TSM-003b ==
  In1 : Inport
  guarantee : Outport  OutDataTypeStr=boolean
  wires:
  In1/1 -> guarantee/1

== system triplex_12B_with_contracts/triplex_12B_TriplexSignalMonitorSpec/TSM-003c ==
  In1 : Inport
  guarantee : Outport  OutDataTypeStr=boolean
  wires:
  In1/1 -> guarantee/1

== system triplex_12B_with_contracts/triplex_12B_TriplexSignalMonitorSpec/TSM-004 ==
  In1 : Inport
  guarantee : Outport  OutDataTypeStr=boolean
  wires:
  In1/1 -> guarantee/1

== system triplex_12B_with_contracts/triplex_12B_TriplexSignalMonitorSpec/abs_call ==
  abs_x : Inport  OutDataTypeStr=double
  branch_6_IF : Switch  Criteria=u2 ~= 0
  xxabs_1_operator : RelationalOperator  OutDataTypeStr=boolean  RndMeth=Simplest
  xxabs_1_rhs_2 : Constant  Value=0.0  OutDataTypeStr=double
  xxabs_2_operator : Gain  Gain=-1  OutDataTypeStr=double
  abs_y : Outport
  wires:
  branch_6_IF/1 -> abs_y/1
  xxabs_1_rhs_2/1 -> xxabs_1_operator/2
  xxabs_2_operator/1 -> branch_6_IF/3
  xxabs_1_operator/1 -> branch_6_IF/2
  abs_x/1 -> xxabs_2_operator/1, xxabs_1_operator/1, branch_6_IF/1

== system triplex_12B_with_contracts/triplex_12B_TriplexSignalMonitorSpec/abs_call1 ==
  abs_x : Inport  OutDataTypeStr=double
  branch_6_IF : Switch  Criteria=u2 ~= 0
  xxabs_1_operator : RelationalOperator  OutDataTypeStr=boolean  RndMeth=Simplest
  xxabs_1_rhs_2 : Constant  Value=0.0  OutDataTypeStr=double
  xxabs_2_operator : Gain  Gain=-1  OutDataTypeStr=double
  abs_y : Outport
  wires:
  branch_6_IF/1 -> abs_y/1
  xxabs_1_rhs_2/1 -> xxabs_1_operator/2
  xxabs_2_operator/1 -> branch_6_IF/3
  xxabs_1_operator/1 -> branch_6_IF/2
  abs_x/1 -> xxabs_2_operator/1, xxabs_1_operator/1, branch_6_IF/1

== system triplex_12B_with_contracts/triplex_12B_TriplexSignalMonitorSpec/abs_call11 ==
  abs_x : Inport  OutDataTypeStr=double
  branch_6_IF : Switch  Criteria=u2 ~= 0
  xxabs_1_operator : RelationalOperator  OutDataTypeStr=boolean  RndMeth=Simplest
  xxabs_1_rhs_2 : Constant  Value=0.0  OutDataTypeStr=double
  xxabs_2_operator : Gain  Gain=-1  OutDataTypeStr=double
  abs_y : Outport
  wires:
  branch_6_IF/1 -> abs_y/1
  xxabs_1_rhs_2/1 -> xxabs_1_operator/2
  xxabs_2_operator/1 -> branch_6_IF/3
  xxabs_1_operator/1 -> branch_6_IF/2
  abs_x/1 -> xxabs_2_operator/1, xxabs_1_operator/1, branch_6_IF/1

== system triplex_12B_with_contracts/TriplexMonitorNoFail/Actions/Act1 ==
  note: // Action 1: No pending failures
  state : Inport
  Action Port : ActionPort  ActionPortLabel=if { }
  Constant1 : Constant  Value=0  OutDataTypeStr=int32
  Demux : Demux  Outputs=3
  Mux : Mux  Inputs=3
  Signal Conversion : SignalConversion  OverrideOpt=off
  Terminator : Terminator
  NextState : Outport  VectorParamsAs1DForOutWhenUnconnected=off
  wires:
  state/1 -> [state]
  Signal Conversion/1 -> NextState/1
  Mux/1 -> Signal Conversion/1
  [state] -> Demux/1
  Demux/2 -> Mux/2
  Demux/3 -> Mux/3
  Constant1/1 -> Mux/1
  Demux/1 -> Terminator/1

== system triplex_12B_with_contracts/TriplexMonitorNoFail/Actions/Act2 ==
  note: // Action 2: Failure pending but no miscompares
  state : Inport
  Action Port : ActionPort  ActionPortLabel=elseif { }
  Constant1 : Constant  OutDataTypeStr=int32
  Demux : Demux  Outputs=3
  Mux : Mux  Inputs=3
  Signal Conversion : SignalConversion  OverrideOpt=off
  Sum : Sum  Inputs=-+|
  NextState : Outport  VectorParamsAs1DForOutWhenUnconnected=off
  wires:
  state/1 -> [state]
  Constant1/1 -> Sum/1
  Signal Conversion/1 -> NextState/1
  Mux/1 -> Signal Conversion/1
  [state] -> Demux/1
  Demux/2 -> Mux/2
  Demux/3 -> Mux/3
  Sum/1 -> Mux/1
  Demux/1 -> Sum/2

== system triplex_12B_with_contracts/TriplexMonitorNoFail/Actions/Act3 ==
  note: // Action 3: Do nothing there is only 1 miscompare
  state : Inport
  Action Port : ActionPort  ActionPortLabel=elseif { }
  NextState : Outport  VectorParamsAs1DForOutWhenUnconnected=off
  wires:
  state/1 -> NextState/1

== system triplex_12B_with_contracts/TriplexMonitorNoFail/Actions/Act4 ==
  note: // Action 4: Failure pending
  state : Inport
  Action Port : ActionPort  ActionPortLabel=elseif { }
  Constant1 : Constant  OutDataTypeStr=int32
  Demux : Demux  Outputs=3
  Mux : Mux  Inputs=3
  Signal Conversion : SignalConversion  OverrideOpt=off
  Sum : Sum  Inputs=++|
  Sum1 : Sum  Inputs=|++
  NextState : Outport  VectorParamsAs1DForOutWhenUnconnected=off
  wires:
  state/1 -> [state]
  Signal Conversion/1 -> NextState/1
  Mux/1 -> Signal Conversion/1
  [state] -> Demux/1
  Demux/2 -> Sum/2
  Constant1/1 -> Sum1/2, Sum/1
  Demux/1 -> Sum1/1
  Sum1/1 -> Mux/1
  Sum/1 -> Mux/2
  Demux/3 -> Mux/3

== system triplex_12B_with_contracts/TriplexMonitorNoFail/Actions/Act5 ==
  note: // Action 5: Failure latched (branch B)
  state : Inport
  Action Port : ActionPort  ActionPortLabel=elseif { }
  Constant : Constant  Value=0  OutDataTypeStr=int32
  Constant1 : Constant  Value=2  OutDataTypeStr=int32
  Mux : Mux  Inputs=3
  Selector : Selector  InputPortWidth=3  IndexOptions=Index vector (dialog)  Indices=[2]  OutputSizes=1
  Signal Conversion : SignalConversion  OverrideOpt=off
  NextState : Outport  VectorParamsAs1DForOutWhenUnconnected=off
  wires:
  state/1 -> [state]
  Mux/1 -> Signal Conversion/1
  Constant/1 -> Mux/1
  Constant1/1 -> Mux/3
  Selector/1 -> Mux/2
  [state] -> Selector/1
  Signal Conversion/1 -> NextState/1

== system triplex_12B_with_contracts/TriplexMonitorNoFail/Actions/Act6 ==
  note: // Action 6: Failure latched (branch A)
  state : Inport
  Action Port : ActionPort  ActionPortLabel=elseif { }
  Constant : Constant  Value=0  OutDataTypeStr=int32
  Constant1 : Constant  Value=4  OutDataTypeStr=int32
  Mux : Mux  Inputs=3
  Selector : Selector  InputPortWidth=3  IndexOptions=Index vector (dialog)  Indices=[2]  OutputSizes=1
  Signal Conversion : SignalConversion  OverrideOpt=off
  NextState : Outport  VectorParamsAs1DForOutWhenUnconnected=off
  wires:
  state/1 -> [state]
  Mux/1 -> Signal Conversion/1
  Constant/1 -> Mux/1
  Constant1/1 -> Mux/3
  Selector/1 -> Mux/2
  [state] -> Selector/1
  Signal Conversion/1 -> NextState/1

== system triplex_12B_with_contracts/TriplexMonitorNoFail/Actions/Act7 ==
  note: /// Action 7: Failure latched (branch C)
  state : Inport
  Action Port : ActionPort  ActionPortLabel=elseif { }
  Constant : Constant  Value=0  OutDataTypeStr=int32
  Constant1 : Constant  OutDataTypeStr=int32
  Mux : Mux  Inputs=3
  Selector : Selector  InputPortWidth=3  IndexOptions=Index vector (dialog)  Indices=[2]  OutputSizes=1
  Signal Conversion : SignalConversion  OverrideOpt=off
  NextState : Outport  VectorParamsAs1DForOutWhenUnconnected=off
  wires:
  state/1 -> [state]
  Mux/1 -> Signal Conversion/1
  Constant/1 -> Mux/1
  Constant1/1 -> Mux/3
  Selector/1 -> Mux/2
  [state] -> Selector/1
  Signal Conversion/1 -> NextState/1

== system triplex_12B_with_contracts/TriplexMonitorNoFail/Actions/Act8 ==
  note: // Action 8: All branches miscompare
  state : Inport
  Action Port : ActionPort  ActionPortLabel=elseif { }
  Constant1 : Constant  OutDataTypeStr=int32
  Demux : Demux  Outputs=3
  Mux : Mux  Inputs=3
  Signal Conversion : SignalConversion  OverrideOpt=off
  Sum1 : Sum  Inputs=++|
  NextState : Outport  VectorParamsAs1DForOutWhenUnconnected=off
  wires:
  state/1 -> [state]
  Mux/1 -> Signal Conversion/1
  Demux/1 -> Mux/1
  Demux/3 -> Mux/3
  Sum1/1 -> Mux/2
  Constant1/1 -> Sum1/1
  Demux/2 -> Sum1/2
  Signal Conversion/1 -> NextState/1
  [state] -> Demux/1

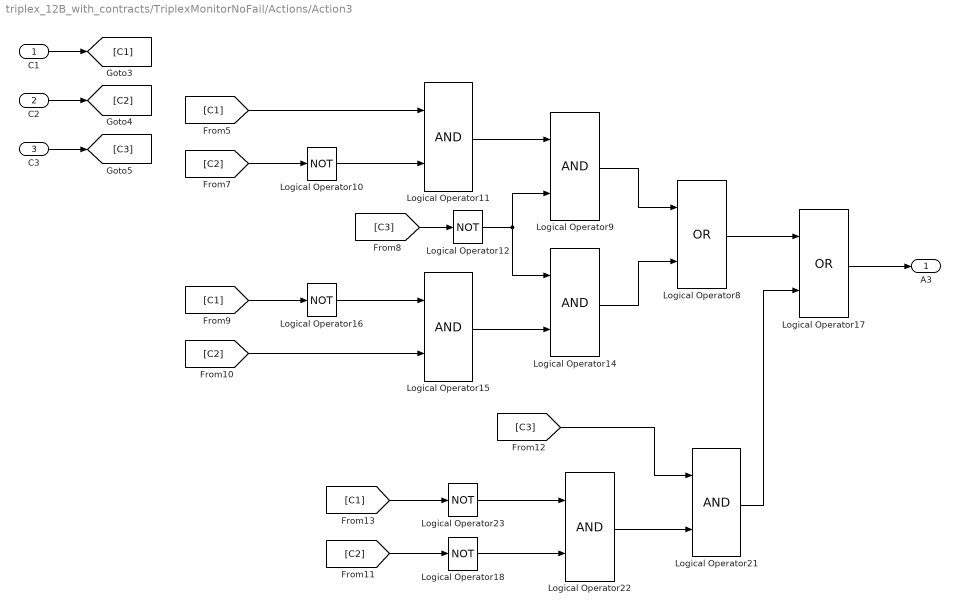
== system triplex_12B_with_contracts/TriplexMonitorNoFail/Actions/Action3 ==
  C1 : Inport
  C2 : Inport  Port=2
  C3 : Inport  Port=3
  Logical Operator{10,12,16,18,23} (5 alike) : Logic  Operator=NOT  Inputs=1  AllPortsSameDT=off  OutDataTypeStr=boolean
  Logical Operator{9,11,14..15,21..22} (6 alike) : Logic  AllPortsSameDT=off  OutDataTypeStr=boolean
  Logical Operator17 : Logic  Operator=OR  AllPortsSameDT=off  OutDataTypeStr=boolean
  Logical Operator8 : Logic  Operator=OR  AllPortsSameDT=off  OutDataTypeStr=boolean
  A3 : Outport  VectorParamsAs1DForOutWhenUnconnected=off
  wires:
  [C1] -> Logical Operator11/1
  [C2] -> Logical Operator10/1
  Logical Operator10/1 -> Logical Operator11/2
  Logical Operator12/1 -> Logical Operator9/2, Logical Operator14/1
  [C3] -> Logical Operator12/1
  Logical Operator11/1 -> Logical Operator9/1
  Logical Operator16/1 -> Logical Operator15/1
  [C1] -> Logical Operator16/1
  Logical Operator9/1 -> Logical Operator8/1
  [C2] -> Logical Operator15/2
  Logical Operator15/1 -> Logical Operator14/2
  Logical Operator14/1 -> Logical Operator8/2
  Logical Operator8/1 -> Logical Operator17/1
  Logical Operator21/1 -> Logical Operator17/2
  [C2] -> Logical Operator18/1
  [C1] -> Logical Operator23/1
  [C3] -> Logical Operator21/1
  Logical Operator23/1 -> Logical Operator22/1
  Logical Operator22/1 -> Logical Operator21/2
  Logical Operator18/1 -> Logical Operator22/2
  Logical Operator17/1 -> A3/1
  C1/1 -> [C1]
  C2/1 -> [C2]
  C3/1 -> [C3]

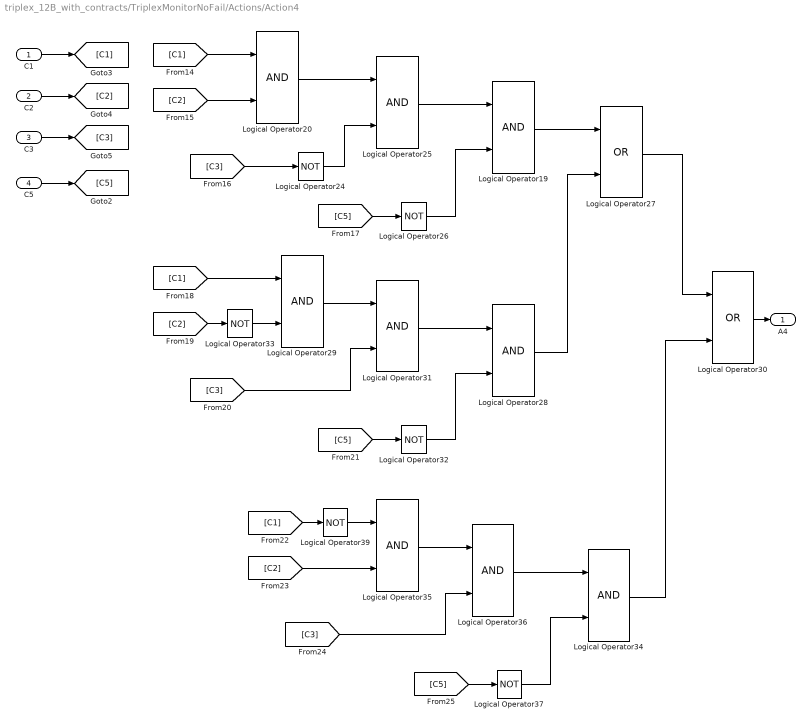
== system triplex_12B_with_contracts/TriplexMonitorNoFail/Actions/Action4 ==
  C1 : Inport
  C2 : Inport  Port=2
  C3 : Inport  Port=3
  C5 : Inport  Port=4
  Logical Operator{19..20,25,28..29,31,34..36} (9 alike) : Logic  AllPortsSameDT=off  OutDataTypeStr=boolean
  Logical Operator{24,26,32..33,37,39} (6 alike) : Logic  Operator=NOT  Inputs=1  AllPortsSameDT=off  OutDataTypeStr=boolean
  Logical Operator27 : Logic  Operator=OR  AllPortsSameDT=off  OutDataTypeStr=boolean
  Logical Operator30 : Logic  Operator=OR  AllPortsSameDT=off  OutDataTypeStr=boolean
  A4 : Outport  VectorParamsAs1DForOutWhenUnconnected=off
  wires:
  [C3] -> Logical Operator31/2
  Logical Operator31/1 -> Logical Operator28/1
  [C5] -> Logical Operator32/1
  Logical Operator32/1 -> Logical Operator28/2
  [C1] -> Logical Operator29/1
  Logical Operator28/1 -> Logical Operator27/2
  Logical Operator29/1 -> Logical Operator31/1
  [C2] -> Logical Operator33/1
  [C3] -> Logical Operator24/1
  [C2] -> Logical Operator20/2
  [C1] -> Logical Operator20/1
  Logical Operator20/1 -> Logical Operator25/1
  Logical Operator30/1 -> A4/1
  Logical Operator26/1 -> Logical Operator19/2
  Logical Operator33/1 -> Logical Operator29/2
  Logical Operator25/1 -> Logical Operator19/1
  [C5] -> Logical Operator26/1
  Logical Operator19/1 -> Logical Operator27/1
  Logical Operator24/1 -> Logical Operator25/2
  Logical Operator36/1 -> Logical Operator34/1
  Logical Operator27/1 -> Logical Operator30/1
  Logical Operator37/1 -> Logical Operator34/2
  [C5] -> Logical Operator37/1
  [C3] -> Logical Operator36/2
  Logical Operator39/1 -> Logical Operator35/1
  Logical Operator35/1 -> Logical Operator36/1
  [C1] -> Logical Operator39/1
  Logical Operator34/1 -> Logical Operator30/2
  [C2] -> Logical Operator35/2
  C1/1 -> [C1]
  C5/1 -> [C5]
  C2/1 -> [C2]
  C3/1 -> [C3]

== system triplex_12B_with_contracts/TriplexMonitorNoFail/Actions/Action8 ==
  C1 : Inport
  C2 : Inport  Port=2
  C3 : Inport  Port=3
  Logical Operator3 : Logic  AllPortsSameDT=off  OutDataTypeStr=boolean
  Logical Operator4 : Logic  AllPortsSameDT=off  OutDataTypeStr=boolean
  A8 : Outport  VectorParamsAs1DForOutWhenUnconnected=off
  wires:
  Logical Operator3/1 -> Logical Operator4/1
  C3/1 -> Logical Operator4/2
  C1/1 -> Logical Operator3/1
  C2/1 -> Logical Operator3/2
  Logical Operator4/1 -> A8/1

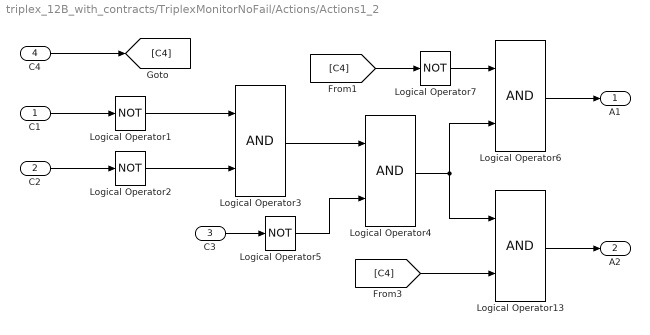
== system triplex_12B_with_contracts/TriplexMonitorNoFail/Actions/Actions1_2 ==
  C1 : Inport
  C2 : Inport  Port=2
  C3 : Inport  Port=3
  C4 : Inport  Port=4
  Logical Operator{1..2,5,7} (4 alike) : Logic  Operator=NOT  Inputs=1  AllPortsSameDT=off  OutDataTypeStr=boolean
  Logical Operator{3..4,6,13} (4 alike) : Logic  AllPortsSameDT=off  OutDataTypeStr=boolean
  A1 : Outport  VectorParamsAs1DForOutWhenUnconnected=off
  A2 : Outport  Port=2  VectorParamsAs1DForOutWhenUnconnected=off
  wires:
  C2/1 -> Logical Operator2/1
  Logical Operator4/1 -> Logical Operator6/2, Logical Operator13/1
  Logical Operator2/1 -> Logical Operator3/2
  [C4] -> Logical Operator13/2
  C1/1 -> Logical Operator1/1
  Logical Operator1/1 -> Logical Operator3/1
  Logical Operator6/1 -> A1/1
  Logical Operator7/1 -> Logical Operator6/1
  Logical Operator3/1 -> Logical Operator4/1
  [C4] -> Logical Operator7/1
  Logical Operator13/1 -> A2/1
  Logical Operator5/1 -> Logical Operator4/2
  C3/1 -> Logical Operator5/1
  C4/1 -> [C4]

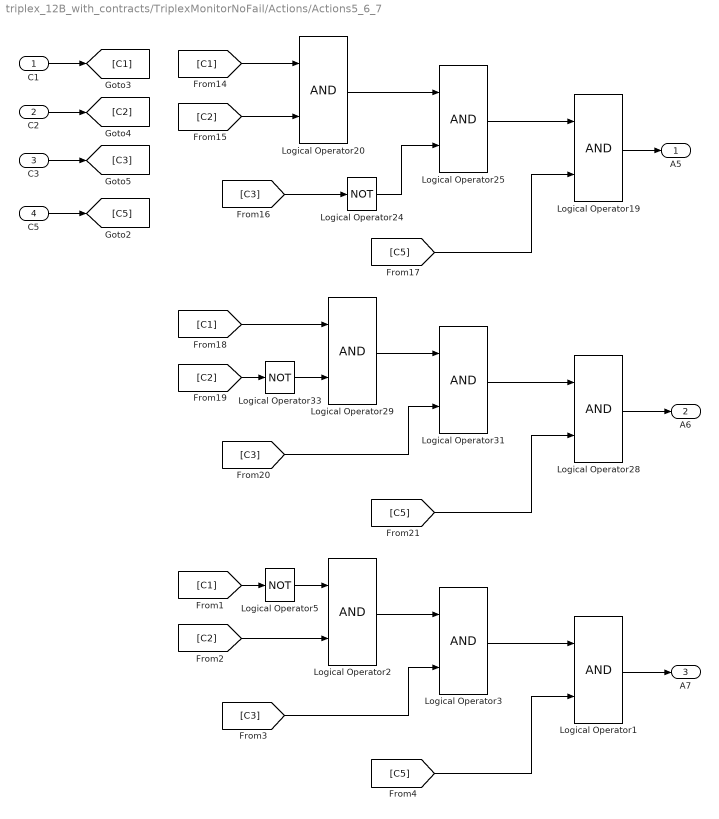
== system triplex_12B_with_contracts/TriplexMonitorNoFail/Actions/Actions5_6_7 ==
  C1 : Inport
  C2 : Inport  Port=2
  C3 : Inport  Port=3
  C5 : Inport  Port=4
  Logical Operator{1..3,19..20,25,28..29,31} (9 alike) : Logic  AllPortsSameDT=off  OutDataTypeStr=boolean
  Logical Operator24 : Logic  Operator=NOT  Inputs=1  AllPortsSameDT=off  OutDataTypeStr=boolean
  Logical Operator33 : Logic  Operator=NOT  Inputs=1  AllPortsSameDT=off  OutDataTypeStr=boolean
  Logical Operator5 : Logic  Operator=NOT  Inputs=1  AllPortsSameDT=off  OutDataTypeStr=boolean
  A5 : Outport  VectorParamsAs1DForOutWhenUnconnected=off
  A6 : Outport  Port=2  VectorParamsAs1DForOutWhenUnconnected=off
  A7 : Outport  Port=3  VectorParamsAs1DForOutWhenUnconnected=off
  wires:
  [C3] -> Logical Operator31/2
  Logical Operator31/1 -> Logical Operator28/1
  [C5] -> Logical Operator28/2
  [C1] -> Logical Operator29/1
  Logical Operator29/1 -> Logical Operator31/1
  [C2] -> Logical Operator33/1
  [C3] -> Logical Operator24/1
  [C2] -> Logical Operator20/2
  [C1] -> Logical Operator20/1
  Logical Operator20/1 -> Logical Operator25/1
  [C5] -> Logical Operator19/2
  Logical Operator33/1 -> Logical Operator29/2
  Logical Operator25/1 -> Logical Operator19/1
  Logical Operator24/1 -> Logical Operator25/2
  C1/1 -> [C1]
  C5/1 -> [C5]
  C2/1 -> [C2]
  C3/1 -> [C3]
  Logical Operator19/1 -> A5/1
  Logical Operator28/1 -> A6/1
  [C3] -> Logical Operator3/2
  Logical Operator3/1 -> Logical Operator1/1
  [C5] -> Logical Operator1/2
  [C1] -> Logical Operator5/1
  Logical Operator2/1 -> Logical Operator3/1
  [C2] -> Logical Operator2/2
  Logical Operator1/1 -> A7/1
  Logical Operator5/1 -> Logical Operator2/1

== system triplex_12B_with_contracts/TriplexMonitorNoFail/Output/No-Fail ==
  note: // Action 1: no-fail state
  ia : Inport
  ib : Inport  Port=2
  ic : Inport  Port=3
  Action Port : ActionPort  ActionPortLabel=if { }
  Avg3 : Subsystem
  choose : Subsystem
  choose1 : Subsystem
  sel_val : Outport  VectorParamsAs1DForOutWhenUnconnected=off
  wires:
  ia/1 -> [ia]
  ib/1 -> [ib]
  ic/1 -> [ic]
  [ia] -> Avg3/1(i1)
  [ib] -> Avg3/2(i2)
  [ic] -> Avg3/3(i3)
  [ia] -> choose/1(i1)
  Avg3/1(Avg) -> choose1/2(avg), choose/2(avg)
  [ib] -> choose/3(i2)
  choose/1(choice) -> choose1/1(i1)
  [ic] -> choose1/3(i2)
  choose1/1(choice) -> sel_val/1

== system triplex_12B_with_contracts/TriplexMonitorNoFail/Output/Single-BranchA-Fail ==
  note: // Action 4: Single-BranchA-Fail
  ib : Inport
  ic : Inport  Port=2
  Action Port : ActionPort  ActionPortLabel=elseif { }
  Avg2 : Subsystem
  sel_val : Outport  VectorParamsAs1DForOutWhenUnconnected=off
  wires:
  Avg2/1(Avg) -> sel_val/1
  [ic] -> Avg2/2(i2)
  [ib] -> Avg2/1(i1)
  ic/1 -> [ic]
  ib/1 -> [ib]

== system triplex_12B_with_contracts/TriplexMonitorNoFail/Output/Single-BranchB-Fail ==
  note: // Action 3: Single-BranchB-Fail
  ia : Inport
  ic : Inport  Port=2
  Action Port : ActionPort  ActionPortLabel=elseif { }
  Avg2 : Subsystem
  sel_val : Outport  VectorParamsAs1DForOutWhenUnconnected=off
  wires:
  ia/1 -> [ia]
  ic/1 -> [ic]
  [ia] -> Avg2/1(i1)
  [ic] -> Avg2/2(i2)
  Avg2/1(Avg) -> sel_val/1

== system triplex_12B_with_contracts/TriplexMonitorNoFail/Output/Single-BranchC-Fail ==
  note: // Action 2: Single-BranchC-Fail
  ia : Inport
  ib : Inport  Port=2
  Action Port : ActionPort  ActionPortLabel=elseif { }
  Avg2 : Subsystem
  sel_val : Outport  VectorParamsAs1DForOutWhenUnconnected=off
  wires:
  Avg2/1(Avg) -> sel_val/1
  [ib] -> Avg2/2(i2)
  [ia] -> Avg2/1(i1)
  ib/1 -> [ib]
  ia/1 -> [ia]

== system triplex_12B_with_contracts/TriplexMonitorNoFail/Output/No-Fail/Avg3 ==
  i1 : Inport
  i2 : Inport  Port=2
  i3 : Inport  Port=3
  Constant : Constant  Value=3.0
  Divide : Product  Inputs=*/
  Sum : Sum  Inputs=|++
  Sum1 : Sum  Inputs=|++
  Avg : Outport  VectorParamsAs1DForOutWhenUnconnected=off
  wires:
  Sum1/1 -> Divide/1
  Constant/1 -> Divide/2
  i2/1 -> Sum/2
  Sum/1 -> Sum1/1
  Divide/1 -> Avg/1
  i3/1 -> Sum1/2
  i1/1 -> Sum/1

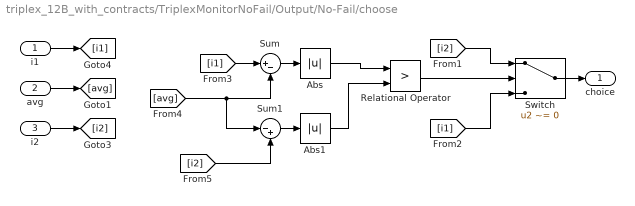
== system triplex_12B_with_contracts/TriplexMonitorNoFail/Output/No-Fail/choose ==
  i1 : Inport
  avg : Inport  Port=2
  i2 : Inport  Port=3
  Abs : Abs
  Abs1 : Abs
  Relational Operator : RelationalOperator  Operator=>  OutDataTypeStr=boolean  RndMeth=Nearest
  Sum : Sum  Inputs=|+-
  Sum1 : Sum  Inputs=|-+
  Switch : Switch  Criteria=u2 ~= 0
  choice : Outport  VectorParamsAs1DForOutWhenUnconnected=off
  wires:
  Abs/1 -> Relational Operator/1
  Switch/1 -> choice/1
  [i1] -> Sum/1
  [i1] -> Switch/3
  [i2] -> Switch/1
  Abs1/1 -> Relational Operator/2
  Sum1/1 -> Abs1/1
  Relational Operator/1 -> Switch/2
  [i2] -> Sum1/2
  Sum/1 -> Abs/1
  [avg] -> Sum1/1, Sum/2
  i1/1 -> [i1]
  avg/1 -> [avg]
  i2/1 -> [i2]
